simulink model "Memresistor"  (R2023a)
settings: Solver=VariableStepAuto  StartTime=0  StopTime=5  RelTol=1e-3
model workspace (MAT data in the model file):
  R1 = 20
  R1_ = 0
  R2 = 500
  VT = 0.5
  a = 500
  b = 1000
settings Model: Creator=Wang Xishengshun  LastModifiedBy=Wang Xishengshun

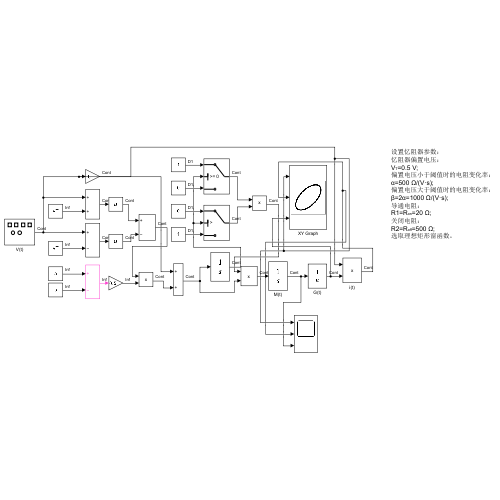
[thumbnail: Simulink's stored preview of the top-level diagram]
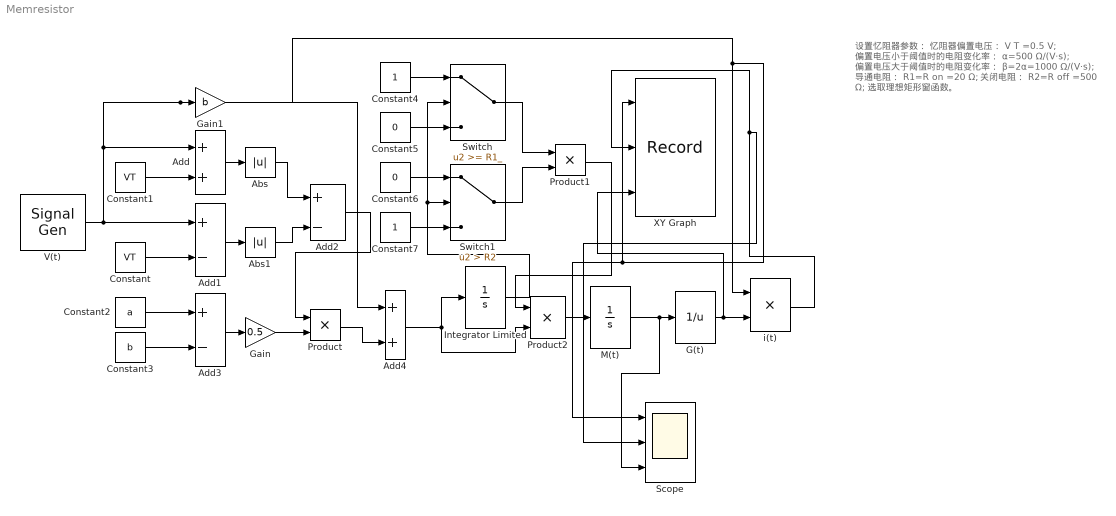
== system Memresistor ==
  note: 设置忆阻器参数：
      | 忆阻器偏置电压：
      | V T =0.5 V;
      | 偏置电压小于阈值时的电阻变化率：
      | α=500 Ω/(V·s);
      | 偏置电压大于阈值时的电阻变化率：
      | β=2α=1000 Ω/(V·s);
      | 导通电阻：
      | R1=R on =20 Ω;
      | 关闭电阻：
      | R2=R off =500 Ω;
      | 选取理想矩形窗函数。
  Abs : Abs  SaturateOnIntegerOverflow=off
  Abs1 : Abs  SaturateOnIntegerOverflow=off
  Add : Sum
  Add1 : Sum  Inputs=+-
  Add2 : Sum  Inputs=+-
  Add3 : Sum  Inputs=+-
  Add4 : Sum
  Constant : Constant  Value=VT
  Constant1 : Constant  Value=VT
  Constant2 : Constant  Value=a
  Constant3 : Constant  Value=b
  Constant4 : Constant  SampleTime=0.01
  Constant5 : Constant  Value=0  SampleTime=0.01
  Constant6 : Constant  Value=0  SampleTime=0.01
  Constant7 : Constant  SampleTime=0.01
  G(t) : Math  Operator=reciprocal
  Gain : Gain  Gain=0.5
  Gain1 : Gain  Gain=b
  Integrator Limited : Integrator  UpperSaturationLimit=1600  LowerSaturationLimit=0  WrappedStateUpperValue=500  WrappedStateLowerValue=0
  M(t) : Integrator  InitialCondition=480  UpperSaturationLimit=1600  LowerSaturationLimit=0  WrappedStateUpperValue=500  WrappedStateLowerValue=0
  Product : Product
  Product1 : Product
  Product2 : Product
  Scope : Scope  NumInputPorts=3
  Switch : Switch  Threshold=R1_  RndMeth=Ceiling  SaturateOnIntegerOverflow=off  InputSameDT=off
  Switch1 : Switch  Criteria=u2 > Threshold  Threshold=R2  RndMeth=Ceiling  SaturateOnIntegerOverflow=off  InputSameDT=off
  V(t) : SignalGenerator  Amplitude=2
  XY Graph : Record  FileSettingsInternal="{\"entries\":[{\"content\":{\"excelSettings\":{\"content\":{},\"type\":\"Streamout.ExcelSettings\"}},\"type\":\"Streamout.FileSettingStorage\",\"uuid\":\"\"}],\"packageUris\":[\"http:\\/\\/schema.mathworks.com\\/mf0\\/streamout_blocks\\/R2020a\"],\"version\":\"1.0\"}"  Layout=[1 2]  SignalsInternal="{\"entries\":[{\"content\":{\"signals\":[{\"content\":{\"blockPath\":[],\"dimensions\":[1],\"domain\":\"\",\"lineColor\":\"#a2142f\",\"plots\":[1,9],\"port\":1,\"sid\":[\"\"],\"signalID\":731,\"signalName\":\"V(t)\"},\"type\":\"RecordBlkView.Signal\",\"uuid\":\"\"},{\"content\":{\"blockPath\":[],\"dimensions\":[1],\"domain\":\"\",\"lineColor\":\"#139fff\",\"plots\":[9],\"port\":2,\"sid\":[\"\"],\"signalID\":735,\"signalName\":\"i(t)\"},\"type\":\"RecordBlkView.Signal\",\"uuid\":\"\"},{\"content\":{\"blockPath\":[],\"dimensions\":[1],\"domain\":\"\",\"lineColor\":\"#77ac30\",\"plots\":[1],\"port\":3,\"sid\":[\"\"],\"signalID\":739,\"signalName\":\"G(t)\"},\"type\":\"RecordBlkView.Signal\",\"uuid\":\"\"}]},\"type\":\"RecordBlkView.InputSignals\",\"uuid\":\"\"}],\"packageUris\":[\"http:\\/\\/schema.mathworks.com\\/mf0\\/streamout_blocks\\/R2020a\"],\"version\":\"1.0\"}"  VisualizationBindings="{\"xyplotplugin\":{\"info\":[{\"series\":[{\"bindingParametersList\":[{\"parameter\":\"X-Axis\",\"signalID\":731,\"signalName\":\"V(t)\"},{\"parameter\":\"Y-Axis\",\"signalID\":739,\"signalName\":\"G(t)\"}],\"seriesID\":21493}],\"subplotID\":1},{\"series\":[{\"bindingParametersList\":[{\"parameter\":\"X-Axis\",\"signalID\":731,\"signalName\":\"V(t)\"},{\"parameter\":\"Y-Axis\",\"signalID\":735,\"signalName\":\"i(t)\"}],\"seriesID\":41036}],\"subplotID\":9}]}}"  CompatibilityTag=XY
  i(t) : Product
  wires:
  V(t)/1 -> Scope/1, XY Graph/1, i(t)/1, Gain1/1, Add/1, Add1/1
  Constant/1 -> Add1/2
  Constant1/1 -> Add/2
  Constant2/1 -> Add3/1
  Constant3/1 -> Add3/2
  Add3/1 -> Gain/1
  Add/1 -> Abs/1
  Add1/1 -> Abs1/1
  Abs/1 -> Add2/1
  Abs1/1 -> Add2/2
  Gain/1 -> Product/2
  Add2/1 -> Product/1
  Gain1/1 -> Add4/1
  Product/1 -> Add4/2
  Constant4/1 -> Switch/1
  Constant5/1 -> Switch/3
  Constant6/1 -> Switch1/1
  Constant7/1 -> Switch1/3
  Switch1/1 -> Product1/2
  Switch/1 -> Product1/1
  Product1/1 -> Product2/1
  Integrator Limited/1 -> Switch/2, Switch1/2
  Add4/1 -> Product2/2, Integrator Limited/1
  Product2/1 -> M(t)/1
  i(t)/1 -> Scope/2, XY Graph/2
  M(t)/1 -> Scope/3, G(t)/1
  G(t)/1 -> i(t)/2, XY Graph/3
